simulink model "manoeuvreSV_light"  (Simulink 7.5)
settings: Solver=ode45  StartTime=0.0  StopTime=10.0  RelTol=1e-3
settings Model: Creator=paris  LastModifiedBy=paris

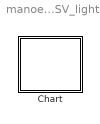
== system manoeuvreSV_light ==
  Chart : Stateflow chart  TreatAsAtomicUnit=on

== stateflow chart Chart ==
  state MANOEUVRESORTIEDEVOIE
    state SVGAUCH
      state HORSDEVOIE
        state Recentration
        state Excentration
        Excentration -> Recentration : [ml.progression_SV==-1]
      state DANSVOIE
      Recentration -> DANSVOIE : [ml.etat_SV==0]
    state IMMINENTE
    (default) -> (junction 10) [order 2] : [ml.lateralisation_SV==-1]
    (default) -> IMMINENTE [order 1] : [ml.tlcCalcule<=1]
    IMMINENTE -> Excentration : [ml.progression_SV==1]
